simulink model "F16lin_K_q"  (R2023b)
settings: Solver=ode4  StartTime=0  StopTime=5  FixedStep=0.01  RelTol=1e-3  EnableMultiTasking=on
values from neighbouring files (symbols this model uses):
  C_l = C_lon(4,:)    [compare_lin_nonlin.m]    (also in plot_Kq_lin_nonlin.m)
  CA_l = C_l*A_lon    [compare_lin_nonlin.m]    (also in plot_Kq_lin_nonlin.m)
  fc = 1/2    (= 0.5)    [compare_lin_nonlin.m]    (also in plot_Kq_lin_nonlin.m)
  invCB_l = inv(CB_l)    [compare_lin_nonlin.m]    (also in plot_Kq_lin_nonlin.m)
  Kq = 2    [compare_lin_nonlin.m]    (also in plot_Kq_lin_nonlin.m)
undefined symbols (not defined in the file or in its folder): A_lon, B_lon, C_lon, D_lon
settings Model: Creator=keviczky  LastModifiedBy=suvo
settings DataIOCC: Decimation=50  SaveFormat=Array  SignalLoggingSaveFormat=ModelDataLogs  ReturnWorkspaceOutputs=off  SignalLoggingName=sigsOut
settings OptimizationCC: BooleanDataType=off
settings DebuggingCC: SaveWithParameterizedLinksMsg=none  UnderspecifiedInitializationDetection=Classic  MergeDetectMultiDrivingBlocksExec=none  SignalResolutionControl=TryResolveAllWithWarning  MultiTaskDSMMsg=warning  MultiTaskCondExecSysMsg=none  UnconnectedInputMsg=warning  UnconnectedOutputMsg=warning  UnconnectedLineMsg=warning
settings HardwareCC: ProdBitPerPointer=32  ProdBitPerSizeT=32  ProdBitPerPtrDiffT=32  ProdLargestAtomicFloat=None  ProdIntDivRoundTo=Undefined  ProdEndianess=Unspecified  ProdWordSize=32  ProdHWDeviceType=32-bit Generic  TargetUnknown=on
settings ModelReferenceCC: PropagateSignalLabelsOutOfModel=off
settings GRTTargetCC: CombineOutputUpdateFcns=off  GRTInterface=on
settings ConfigComp: CovMetricSettings=dw  CovSaveCumulativeToWorkspaceVar=on  CovSaveSingleToWorkspaceVar=on

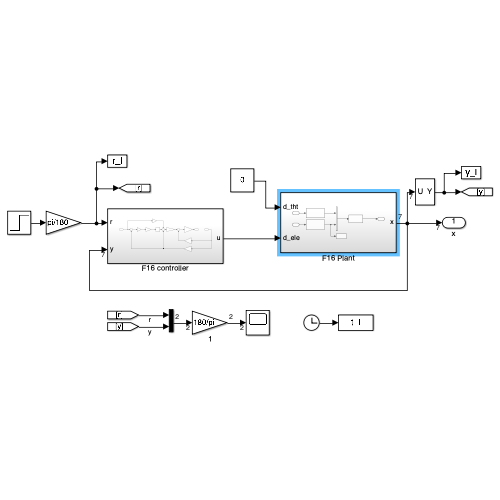
[thumbnail: Simulink's stored preview of the top-level diagram]
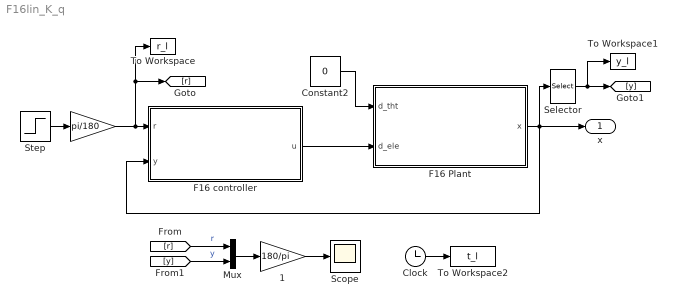
== system F16lin_K_q ==
  " " : Gain  Gain=pi/180
  " 1" : Gain  Gain=180/pi
  Clock : Clock
  Constant2 : Constant  Value=0
  F16 Plant : Subsystem
  F16 controller : Subsystem
  Mux : Mux  Inputs=2
  Scope : Scope
  Selector : Selector  InputPortWidth=7  IndexOptions=Index vector (dialog)  Indices=4  OutputSizes=1
  Step : Step  SampleTime=0
  To Workspace : ToWorkspace  VariableName=r_l  SampleTime=-1
  To Workspace1 : ToWorkspace  VariableName=y_l  SampleTime=-1
  To Workspace2 : ToWorkspace  VariableName=t_l  SampleTime=-1
  x : Outport
  wires:
  Constant2/1 -> F16 Plant/1(d_tht)
  F16 Plant/1(x) -> Selector/1, F16 controller/2(y), x/1
  Step/1 -> " "/1
  F16 controller/1(u) -> F16 Plant/2(d_ele)
  [r] -> Mux/1  "r"
  [y] -> Mux/2  "y"
  Mux/1 -> " 1"/1
  Selector/1 -> To Workspace1/1, [y]
  " "/1 -> F16 controller/1(r), To Workspace/1, [r]
  " 1"/1 -> Scope/1
  Clock/1 -> To Workspace2/1

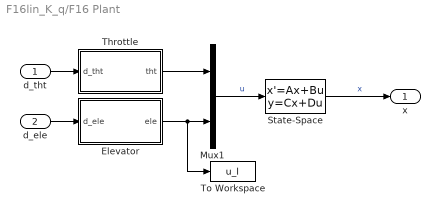
== system F16lin_K_q/F16 Plant ==
  d_tht : Inport
  d_ele : Inport  Port=2
  Elevator : Subsystem
  Mux1 : Mux  Inputs=2
  State-Space : StateSpace  A=A_lon  B=B_lon  C=C_lon  D=D_lon  InitialCondition=0
  Throttle : Subsystem
  To Workspace : ToWorkspace  VariableName=u_l  SampleTime=-1
  x : Outport
  wires:
  d_tht/1 -> Throttle/1(d_tht)
  Mux1/1 -> State-Space/1  "u"
  d_ele/1 -> Elevator/1(d_ele)
  State-Space/1 -> x/1  "x"
  Throttle/1(tht) -> Mux1/1
  Elevator/1(ele) -> To Workspace/1, Mux1/2

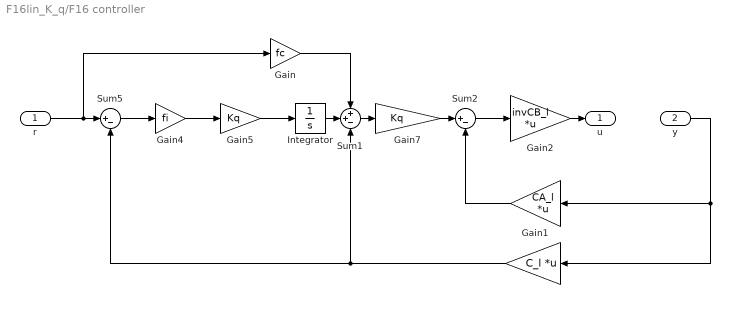
== system F16lin_K_q/F16 controller ==
  r : Inport
  y : Inport  Port=2
  " " : Gain  Gain=C_l  Multiplication=Matrix(K*u)
  Gain : Gain  Gain=fc
  Gain1 : Gain  Gain=CA_l  Multiplication=Matrix(K*u)
  Gain2 : Gain  Gain=invCB_l  Multiplication=Matrix(K*u)
  Gain4 : Gain  Gain=fi
  Gain5 : Gain  Gain=Kq
  Gain7 : Gain  Gain=Kq
  Integrator : Integrator
  Sum1 : Sum  Inputs=++-
  Sum2 : Sum  Inputs=|+-
  Sum5 : Sum  Inputs=|+-
  u : Outport
  wires:
  Gain2/1 -> u/1
  Sum1/1 -> Gain7/1
  r/1 -> Gain/1, Sum5/1
  y/1 -> " "/1, Gain1/1
  Gain5/1 -> Integrator/1
  Sum2/1 -> Gain2/1
  Gain1/1 -> Sum2/2
  Gain/1 -> Sum1/1
  Sum5/1 -> Gain4/1
  Gain4/1 -> Gain5/1
  " "/1 -> Sum5/2, Sum1/3
  Gain7/1 -> Sum2/1
  Integrator/1 -> Sum1/2

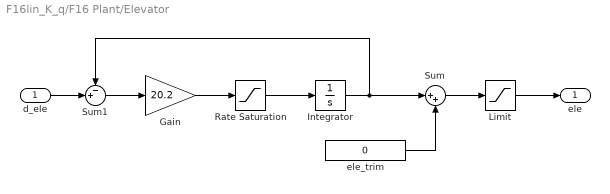
== system F16lin_K_q/F16 Plant/Elevator ==
  d_ele : Inport
  Gain : Gain  Gain=20.2  SaturateOnIntegerOverflow=on  OutDataTypeStr=Inherit: Same as input  ParamDataTypeStr=Inherit: Same as input
  Integrator : Integrator  UpperSaturationLimit=25  LowerSaturationLimit=-25
  Limit : Saturate  UpperLimit=25  LowerLimit=-25
  Rate Saturation : Saturate  UpperLimit=60  LowerLimit=-60
  Sum : Sum  Inputs=|++  InputSameDT=on  SaturateOnIntegerOverflow=on  OutDataTypeStr=Inherit: Same as first input
  Sum1 : Sum  Inputs=-+|  InputSameDT=on  SaturateOnIntegerOverflow=on  OutDataTypeStr=Inherit: Same as first input
  ele_trim : Constant  Value=0
  ele : Outport
  wires:
  Sum1/1 -> Gain/1
  Gain/1 -> Rate Saturation/1
  Rate Saturation/1 -> Integrator/1
  Integrator/1 -> Sum/1, Sum1/1
  Sum/1 -> Limit/1
  Limit/1 -> ele/1
  ele_trim/1 -> Sum/2
  d_ele/1 -> Sum1/2

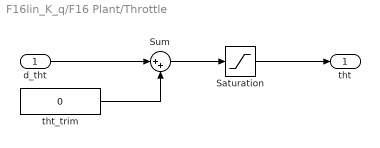
== system F16lin_K_q/F16 Plant/Throttle ==
  d_tht : Inport
  Saturation : Saturate  UpperLimit=1  LowerLimit=0
  Sum : Sum  Inputs=|++  InputSameDT=on  SaturateOnIntegerOverflow=on  OutDataTypeStr=Inherit: Same as first input
  tht_trim : Constant  Value=0
  tht : Outport
  wires:
  Sum/1 -> Saturation/1
  Saturation/1 -> tht/1
  d_tht/1 -> Sum/1
  tht_trim/1 -> Sum/2
